simulink model "system_test"  (R2024b)
settings: Solver=VariableStepAuto  StartTime=0.0  StopTime=10  RelTol=1e-3
values from neighbouring files (symbols this model uses):
  N = NM + mp*diff(x + L*sin(theta),t,2)    [get_k.m]    (also in psoinrmatrix.m = Nm + mp * (x2 + L * (ddtheta * cos(theta) - dtheta ^ 2 * sin; sys_cal.m = Nm+mp*(x2+L*(theta2*cos(theta)-theta1^2*sin(theta))))
undefined symbols (not defined in the file or in its folder): X, Y, Z
libraries: sm_lib x61, nesl_utility x18, slpidlib x1
(part 1 of 3)
settings Model: Creator=PC  LastModifiedBy=admin
settings RTWCC: GPUComputeCapability=3.5

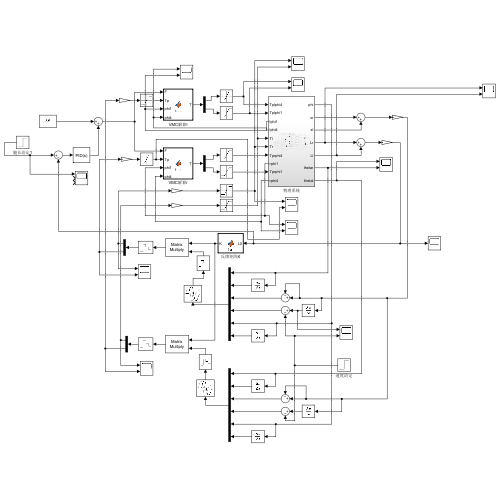
[thumbnail: Simulink's stored preview of the top-level diagram]
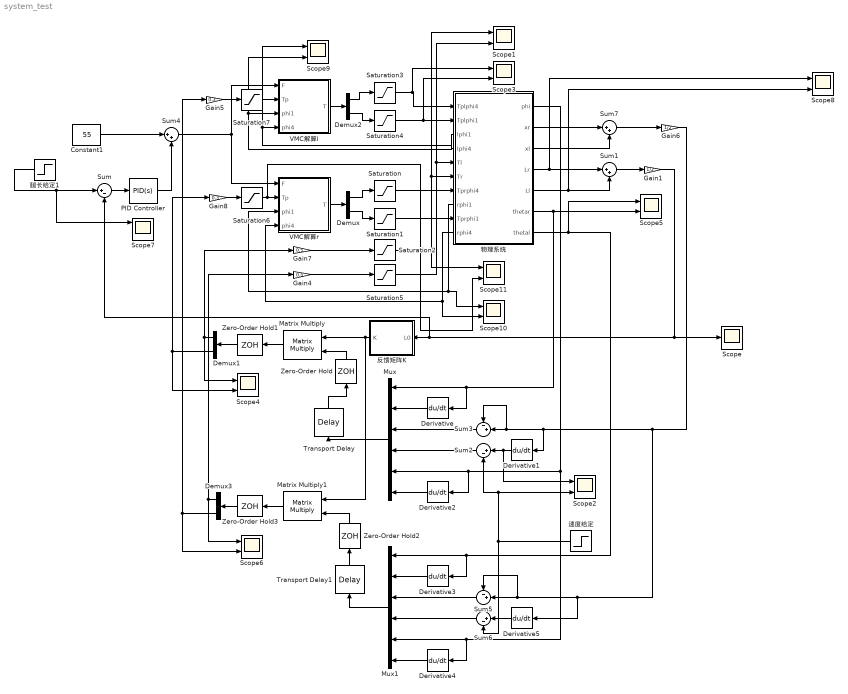
== system system_test ==
  Constant1 : Constant  Value=55
  Demux{,1..3} (4 alike) : Demux  Outputs=2
  Derivative{,1..5} (6 alike) : Derivative
  Gain1 : Gain  Gain=1/2
  Gain4 : Gain  Gain=0.5
  Gain5 : Gain  Gain=0.3
  Gain6 : Gain  Gain=1/2
  Gain7 : Gain  Gain=0.5
  Gain8 : Gain  Gain=0.3
  Matrix Multiply : Product  Multiplication=Matrix(*)
  Matrix Multiply1 : Product  Multiplication=Matrix(*)
  Mux : Mux  Inputs=6
  Mux1 : Mux  Inputs=6
  PID Controller : slpidlib/PID Controller  Controller=PID  Form=Parallel  TimeDomain=Continuous-time  UseExternalTs=off  SampleTime=-1  IntegratorMethod=Forward Euler  FilterMethod=Forward Euler  ControllerParametersSource=internal  P=500  I=0  UseKiTs=off  D=1000  UseExternalDerivativeSource=off  N=100  UseFilter=on  TunerSelectOption=Transfer Function Based (PID Tuner App)  InitialConditionSource=internal  InitialConditionForIntegrator=0  InitialConditionForFilter=0  DifferentiatorICPrevScaledInput=0  ExternalReset=none  TrackingMode=off  Kt=1  LimitOutput=off  SatLimitsSource=internal  UpperSaturationLimit=inf  LowerSaturationLimit=-inf  LinearizeAsGain=on  AntiWindupMode=none  Kb=1  LimitIntegrator=off  UpperIntegratorSaturationLimit=1.5  LowerIntegratorSaturationLimit=-1.5  POutMin=[]  POutMax=[]  IOutMin=[]  IOutMax=[]  DOutMin=[]  DOutMax=[]  NOutMin=[]  NOutMax=[]  SumOutMin=[]  SumOutMax=[]  SaturationOutMin=[]  SaturationOutMax=[]  PParamMin=[]  PParamMax=[]  IParamMin=[]  IParamMax=[]  DParamMin=[]  DParamMax=[]  NParamMin=[]  NParamMax=[]  KbParamMin=[]  KbParamMax=[]  KtParamMin=[]  KtParamMax=[]  KbOutMin=[]  KbOutMax=[]  KtOutMin=[]  KtOutMax=[]  IntegratorOutMin=[]  IntegratorOutMax=[]  FilterOutMin=[]  FilterOutMax=[]  SumI1OutMin=[]  SumI1OutMax=[]  SumI2OutMin=[]  SumI2OutMax=[]  SumI3OutMin=[]  SumI3OutMax=[]  SumI4OutMin=[]  SumI4OutMax=[]  SumDOutMin=[]  SumDOutMax=[]  DifferentiatorOutMin=[]  DifferentiatorOutMax=[]  FilterDiffOutCoefMin=[]  FilterDiffOutCoefMax=[]  ReciprocalOutMin=[]  ReciprocalOutMax=[]  SumDenOutMin=[]  SumDenOutMax=[]  SumNumOutMin=[]  SumNumOutMax=[]  DivideOutMin=[]  DivideOutMax=[]  UdiffTsProdOutMin=[]  UdiffTsProdOutMax=[]  NTsProdOutMin=[]  NTsProdOutMax=[]  UintegralTsProdOutMin=[]  UintegralTsProdOutMax=[]  UngainTsProdOutMin=[]  UngainTsProdOutMax=[]  ClampingZeroOutDataTypeStr=Inherit: Inherit via back propagation  ClampingZeroOutMin=[]  ClampingZeroOutMax=[]  FilterDenConstantOutDataTypeStr=Inherit: Inherit via back propagation  FilterDenConstantOutMin=[]  FilterDenConstantOutMax=[]  PCopyOutDataTypeStr=Inherit: Inherit via back propagation  PCopyOutMin=[]  PCopyOutMax=[]  NCopyOutDataTypeStr=Inherit: Inherit via back propagation  NCopyOutMin=[]  NCopyOutMax=[]  IntegratorContinuousStateAttributes=''  IntegratorStateMustResolveToSignalObject=off  IntegratorRTWStateStorageClass=Auto  FilterContinuousStateAttributes=''  FilterStateMustResolveToSignalObject=off  FilterRTWStateStorageClass=Auto  ParallelPVariant=InternalParameters  IdealPVariant=Disabled  IVariant=InternalParameters  DVariant=InternalParameters  IntegratorVariant=Continuous  SatVariant=Disabled  AWVariant=Passthrough  PCopyVariant=Disabled  TRVariant=Disabled  FdbkBlocksVariant=Forward  IdealPFdbkVariant=Disabled  SatFdbkVariant=Disabled  DerivativeFilterVariant=ContFilter  NVariant=InternalParameters  NCopyVariant=Disabled  FilterICVariant=InternalICsFilter  IntegratorICVariant=InternalICs  ExternalResetVariant=Disabled  TRSumVariant=Passthrough  SumFdbkVariant=Disabled  SumVariant=Sum_PID  TsampFilterVariant=InternalTs  TsampNgainVariant=Passthrough  TsampIntegralVariant=Disabled_SignalSpec  ExternalSaturationOutDataTypeStr=Inherit: Same as second input  DerivativeSourceVariant=ErrorSignal  PreIntVariant=InternalPreInt
  Saturation{,1,3..4} (4 alike) : Saturate  UpperLimit=8  LowerLimit=-8  ZeroCross=off
  Saturation2 : Saturate  UpperLimit=1.2  LowerLimit=-1.2  ZeroCross=off
  Saturation5 : Saturate  UpperLimit=1.2  LowerLimit=-1.2  ZeroCross=off
  Saturation6 : Saturate  UpperLimit=2  LowerLimit=-2  ZeroCross=off
  Saturation7 : Saturate  UpperLimit=2  LowerLimit=-2  ZeroCross=off
  Scope : Scope
  Scope{1..6,8..11} (10 alike) : Scope  NumInputPorts=2
  Scope7 : Scope  NumInputPorts=3
  Sum : Sum  Inputs=|+-
  Sum1 : Sum  Inputs=|++
  Sum2 : Sum  Inputs=|+-
  Sum3 : Sum  Inputs=-+|
  Sum4 : Sum  Inputs=|++
  Sum5 : Sum  Inputs=-+|
  Sum6 : Sum  Inputs=|+-
  Sum7 : Sum  Inputs=|++
  Transport Delay : TransportDelay  DelayTime=0.0000001
  Transport Delay1 : TransportDelay  DelayTime=0.000001
  VMC解算l : MATLAB Function  TreatAsAtomicUnit=on
  VMC解算r : MATLAB Function  TreatAsAtomicUnit=on
  Zero-Order Hold : ZeroOrderHold  SampleTime=0.005
  Zero-Order Hold1 : ZeroOrderHold  SampleTime=0.004
  Zero-Order Hold2 : ZeroOrderHold  SampleTime=0.005
  Zero-Order Hold3 : ZeroOrderHold  SampleTime=0.004
  反馈矩阵K : MATLAB Function  TreatAsAtomicUnit=on
  物理系统 : Subsystem
      settings: PortSchema="{\"entries\":[{\"content\":{\"sides\":[{\"content\":{\"connectorIds\":[\"In1\",\"In2\",\"Out8\",\"Out9\",\"In3\",\"In4\",\"In5\",\"Out10\",\"In6\",\"Out11\"]},\"type\":\"ConnectorPlacement.EquallySpacedRectSide\",\"uuid\":\"664d59a3-0a31-49e2-bbc6-fa33d49ec8c0\"},{\"content\":{\"connectorIds\":[\"Out1\",\"Out2\",\"Out3\",\"Out4\",\"Out5\",\"Out6\",\"Out7\"],\"side\":\"RIGHT\"},\"type\":\"ConnectorPlacement.EquallySpacedRectSide\",\"uuid\":\"d048cd87-328e-45c8-839d-92aa139afc03\"},{\"content\":{\"side\":\"TOP\"},\"type\":\"ConnectorPlacement.EquallySpacedRectSide\",\"uuid\":\"f5424ee2-3185-467c-8de4-9f4b544a14b9\"}]},\"type\":\"ConnectorPlacement.EquallySpacedConnector\",\"uuid\":\"b3bc5ba0-ba30-4936-a275-c2533c1238aa\"}],\"packageUris\":[\"http://schema.mathworks.com/mf0/Connector/R2020b\"],\"version\":\"1.0\"}"
  腿长给定1 : Step  Time=2  Before=0.2  After=0.2  SampleTime=0
  速度给定 : Step  Time=3  After=0.5  SampleTime=0
  wires:
  Sum3/1 -> Mux/3
  Transport Delay/1 -> Zero-Order Hold/1
  物理系统/11(rphi4) -> Scope10/2, VMC解算r/4(phi4)
  Mux/1 -> Transport Delay/1
  Zero-Order Hold/1 -> Matrix Multiply/2
  Derivative1/1 -> Scope2/1, Sum2/1
  Demux/2 -> Saturation1/1
  Saturation/1 -> 物理系统/5(Tprphi4)
  物理系统/6(thetar) -> Derivative/1, Mux/1, Scope5/2
  Demux1/1 -> Gain7/1, Scope4/1
  Derivative2/1 -> Mux/6
  Saturation2/1 -> Scope1/1, 物理系统/4(Tr), Scope11/1
  Sum/1 -> PID Controller/1
  Zero-Order Hold1/1 -> Demux1/1
  Derivative/1 -> Mux/2
  Sum2/1 -> Mux/4
  反馈矩阵K/1(K) -> Matrix Multiply1/1, Matrix Multiply/1
  Matrix Multiply/1 -> Zero-Order Hold1/1
  VMC解算r/1(T) -> Demux/1
  Demux/1 -> Saturation/1
  物理系统/1(phi) -> Derivative4/1, Mux1/5, Mux/5, Derivative2/1
  腿长给定1/1 -> Scope7/1, Sum/1
  Saturation1/1 -> 物理系统/6(Tprphi1)
  物理系统/10(rphi1) -> Scope10/1, VMC解算r/3(phi1)
  Demux1/2 -> Gain8/1, Scope4/2
  PID Controller/1 -> Sum4/2
  Constant1/1 -> Sum4/1
  Sum4/1 -> VMC解算r/1(F), VMC解算l/1(F)
  VMC解算l/1(T) -> Demux2/1
  Demux2/1 -> Saturation3/1
  Demux2/2 -> Saturation4/1
  Saturation4/1 -> Scope3/2, 物理系统/2(Tplphi1)
  Derivative3/1 -> Mux1/2
  Derivative4/1 -> Mux1/6
  物理系统/8(lphi1) -> Scope9/2, VMC解算l/3(phi1)
  物理系统/4(Lr) -> Scope8/1, Sum1/1
  物理系统/5(Ll) -> Scope8/2, Sum1/2
  物理系统/7(thetal) -> Scope5/1, Derivative3/1, Mux1/1
  Sum6/1 -> Mux1/4
  Sum5/1 -> Mux1/3
  Transport Delay1/1 -> Zero-Order Hold2/1
  Mux1/1 -> Transport Delay1/1
  Zero-Order Hold2/1 -> Matrix Multiply1/2
  Matrix Multiply1/1 -> Zero-Order Hold3/1
  Zero-Order Hold3/1 -> Demux3/1
  Sum1/1 -> Gain1/1
  Gain1/1 -> Sum/2, 反馈矩阵K/1(L0), Scope/1
  物理系统/9(lphi4) -> Scope9/1, VMC解算l/4(phi4)
  Demux3/1 -> Scope6/1, Gain4/1
  Saturation5/1 -> Scope1/2, 物理系统/3(Tl)
  Derivative5/1 -> Sum6/1
  Gain4/1 -> Saturation5/1
  Demux3/2 -> Scope6/2, Gain5/1
  Gain5/1 -> Saturation7/1
  速度给定/1 -> Sum6/2, Sum2/2, Scope2/2
  物理系统/2(xr) -> Sum7/1
  物理系统/3(xl) -> Sum7/2
  Sum7/1 -> Gain6/1
  Gain6/1 -> Derivative5/1, Sum5/2, Sum5/1, Derivative1/1, Sum3/1, Sum3/2
  Gain7/1 -> Saturation2/1
  Gain8/1 -> Saturation6/1
  Saturation3/1 -> Scope3/1, 物理系统/1(Tplphi4)
  Saturation6/1 -> Scope11/2, VMC解算r/2(Tp)
  Saturation7/1 -> VMC解算l/2(Tp)
